simulink model "test"  (R2019b)
settings: Solver=FixedStepDiscrete  StartTime=0.0  StopTime=10.0  RelTol=1e-3
values from neighbouring files (symbols this model uses):
  a = getfullname(s_funcs(1))    [instrument_s_functions.m]    (also in test_array.m = [1 2 3 4;5 6 7 8]; test_functions.m = instrument_s_functions(model); test_translates.m = mk{1})
  b = aoe_tsinghua_mhi_data.signals(rp)    [mutate_seed.m]    (also in random_element_from_set.m = ele_set(rp); random_element_from_two_sets.m = r_t_set(rp); test_array.m = 1.4)
settings Model: Creator=yangy  LastModifiedBy=yangy
settings DataIOCC: SaveFormat=Array  SignalLogging=off
settings OptimizationCC: DefaultParameterBehavior=Inlined  EnhancedBackFolding=on  PassReuseOutputArgsThreshold=0  OptimizeBlockOrder=speed  DifferentSizesBufferReuse=on  OptimizationCustomize=off
settings DebuggingCC: ParameterTunabilityLossMsg=error
settings SFSimCC: MATLABDynamicMemAlloc=off
settings RTWCC: Description=Create Visual C/C++ Solution File for Simulink Coder  TemplateMakefile=RTW.MSVCBuild  GenerateReport=on  LaunchReport=on
settings CodeAppCC: ForceParamTrailComments=on  OperatorAnnotations=on

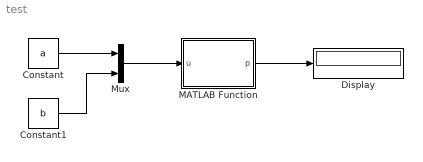
== system test ==
  Constant : Constant  Value=a
  Constant1 : Constant  Value=b
  Display : Display
  MATLAB Function : MATLAB Function  TreatAsAtomicUnit=on
  Mux : Mux  Inputs=2
  wires:
  Constant/1 -> Mux/1
  Constant1/1 -> Mux/2
  Mux/1 -> MATLAB Function/1(u)
  MATLAB Function/1(p) -> Display/1

== matlab function test/MATLAB Function ==
  data: u input; p output
function p  = fcn(u)
    coder.extrinsic('evalin', 'assignin');
%     assignin('base','run_info',strcat(evalin('base','run_info'),'Bd#',sprintf('%f',u(2)),'$'));
    assignin('base','run_info',sprintf('%sBd#%f$',evalin('base','run_info'),u(2)));
    p = 0;
    if u(1) < 50
        p = 40;
    else
        if u(2) == 50
            p = 600;
        end
        p = p + 60;
    end
end
